simulink library "FUSA_FAULTVAIMAN"  (R2024b)
settings: Solver=VariableStepAuto  StartTime=0.0  StopTime=10.0  RelTol=1e-3
undefined symbols (not defined in the file or in its folder): FUSA_AvailState
libraries: simulink x2
settings Model: Creator=jmbsp  LastModifiedBy=jmbsp

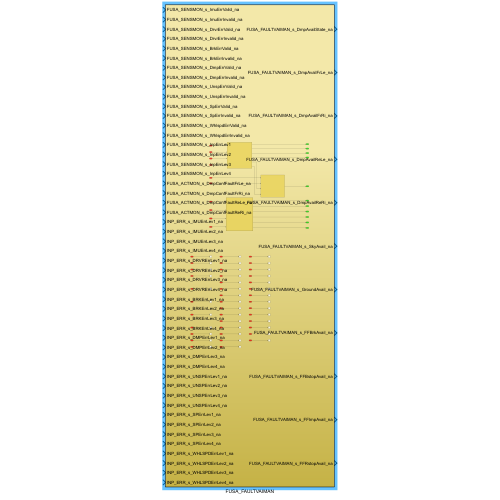
[thumbnail: Simulink's stored preview of the top-level diagram]
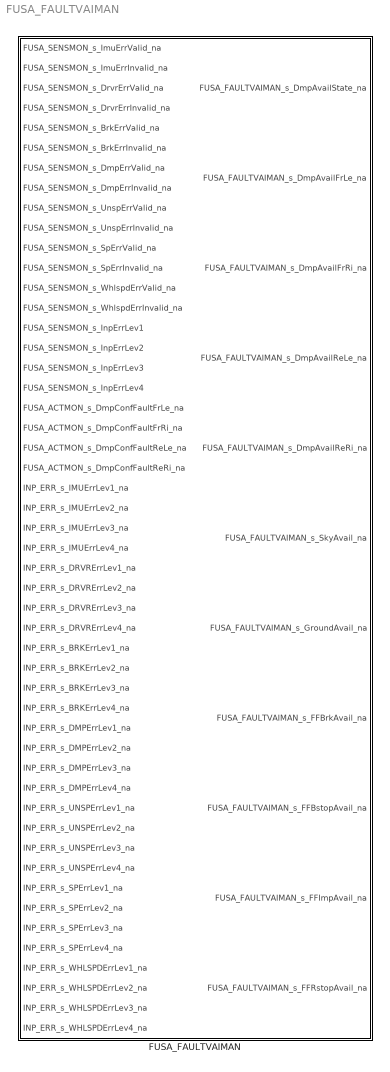
== system FUSA_FAULTVAIMAN ==
  FUSA_FAULTVAIMAN : Subsystem

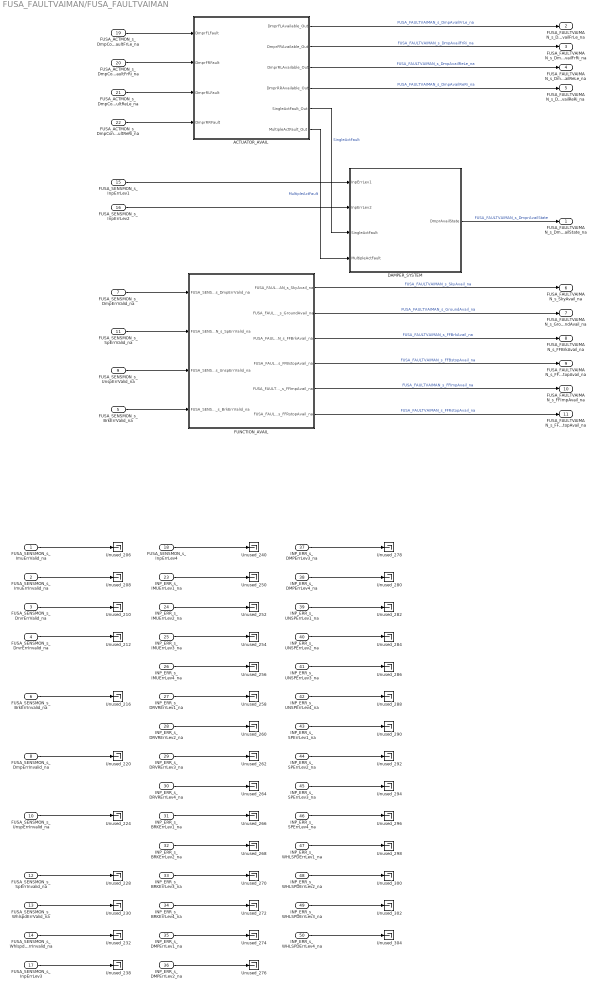
== system FUSA_FAULTVAIMAN/FUSA_FAULTVAIMAN ==
  FUSA_SENSMON_s_ImuErrValid_na : Inport
  FUSA_SENSMON_s_ImuErrInvalid_na : Inport  Port=2
  FUSA_SENSMON_s_DrvrErrValid_na : Inport  Port=3
  FUSA_SENSMON_s_DrvrErrInvalid_na : Inport  Port=4
  FUSA_SENSMON_s_BrkErrValid_na : Inport  Port=5
  FUSA_SENSMON_s_BrkErrInvalid_na : Inport  Port=6
  FUSA_SENSMON_s_DmpErrValid_na : Inport  Port=7
  FUSA_SENSMON_s_DmpErrInvalid_na : Inport  Port=8
  FUSA_SENSMON_s_UnspErrValid_na : Inport  Port=9
  FUSA_SENSMON_s_UnspErrInvalid_na : Inport  Port=10
  FUSA_SENSMON_s_SpErrValid_na : Inport  Port=11
  FUSA_SENSMON_s_SpErrInvalid_na : Inport  Port=12
  FUSA_SENSMON_s_WhlspdErrValid_na : Inport  Port=13
  FUSA_SENSMON_s_WhlspdErrInvalid_na : Inport  Port=14
  FUSA_SENSMON_s_InpErrLev1 : Inport  Port=15  OutDataTypeStr=boolean  PortDimensions=1
  FUSA_SENSMON_s_InpErrLev2 : Inport  Port=16  OutDataTypeStr=boolean  PortDimensions=1
  FUSA_SENSMON_s_InpErrLev3 : Inport  Port=17  OutDataTypeStr=boolean  PortDimensions=1
  FUSA_SENSMON_s_InpErrLev4 : Inport  Port=18  OutDataTypeStr=boolean  PortDimensions=1
  FUSA_ACTMON_s_DmpConfFaultFrLe_na : Inport  Port=19  OutDataTypeStr=boolean  PortDimensions=1
  FUSA_ACTMON_s_DmpConfFaultFrRi_na : Inport  Port=20  OutDataTypeStr=boolean  PortDimensions=1
  FUSA_ACTMON_s_DmpConfFaultReLe_na : Inport  Port=21  OutDataTypeStr=boolean  PortDimensions=1
  FUSA_ACTMON_s_DmpConfFaultReRi_na : Inport  Port=22  OutDataTypeStr=boolean  PortDimensions=1
  INP_ERR_s_IMUErrLev1_na : Inport  Port=23
  INP_ERR_s_IMUErrLev2_na : Inport  Port=24
  INP_ERR_s_IMUErrLev3_na : Inport  Port=25
  INP_ERR_s_IMUErrLev4_na : Inport  Port=26
  INP_ERR_s_DRVRErrLev1_na : Inport  Port=27
  INP_ERR_s_DRVRErrLev2_na : Inport  Port=28
  INP_ERR_s_DRVRErrLev3_na : Inport  Port=29
  INP_ERR_s_DRVRErrLev4_na : Inport  Port=30
  INP_ERR_s_BRKErrLev1_na : Inport  Port=31
  INP_ERR_s_BRKErrLev2_na : Inport  Port=32
  INP_ERR_s_BRKErrLev3_na : Inport  Port=33
  INP_ERR_s_BRKErrLev4_na : Inport  Port=34
  INP_ERR_s_DMPErrLev1_na : Inport  Port=35
  INP_ERR_s_DMPErrLev2_na : Inport  Port=36
  INP_ERR_s_DMPErrLev3_na : Inport  Port=37
  INP_ERR_s_DMPErrLev4_na : Inport  Port=38
  INP_ERR_s_UNSPErrLev1_na : Inport  Port=39
  INP_ERR_s_UNSPErrLev2_na : Inport  Port=40
  INP_ERR_s_UNSPErrLev3_na : Inport  Port=41
  INP_ERR_s_UNSPErrLev4_na : Inport  Port=42
  INP_ERR_s_SPErrLev1_na : Inport  Port=43
  INP_ERR_s_SPErrLev2_na : Inport  Port=44
  INP_ERR_s_SPErrLev3_na : Inport  Port=45
  INP_ERR_s_SPErrLev4_na : Inport  Port=46
  INP_ERR_s_WHLSPDErrLev1_na : Inport  Port=47
  INP_ERR_s_WHLSPDErrLev2_na : Inport  Port=48
  INP_ERR_s_WHLSPDErrLev3_na : Inport  Port=49
  INP_ERR_s_WHLSPDErrLev4_na : Inport  Port=50
  ACTUATOR_AVAIL : Subsystem
  DAMPER_SYSTEM : Subsystem
  FUNCTION_AVAIL : Subsystem
  Unused_{206,208,210,212,216,220,224,228,230,232,238,240,250,252,254,256,258,260,262,264,266,268,270,272,274,276,278,280,282,284,286,288,290,292,294,296,298,300,302,304} (40 alike) : Terminator
  FUSA_FAULTVAIMAN_s_DmpAvailState_na : Outport  OutDataTypeStr=Enum: FUSA_AvailState
  FUSA_FAULTVAIMAN_s_DmpAvailFrLe_na : Outport  Port=2  OutDataTypeStr=boolean
  FUSA_FAULTVAIMAN_s_DmpAvailFrRi_na : Outport  Port=3  OutDataTypeStr=boolean
  FUSA_FAULTVAIMAN_s_DmpAvailReLe_na : Outport  Port=4  OutDataTypeStr=boolean
  FUSA_FAULTVAIMAN_s_DmpAvailReRi_na : Outport  Port=5  OutDataTypeStr=boolean
  FUSA_FAULTVAIMAN_s_SkyAvail_na : Outport  Port=6  OutDataTypeStr=boolean
  FUSA_FAULTVAIMAN_s_GroundAvail_na : Outport  Port=7  OutDataTypeStr=boolean
  FUSA_FAULTVAIMAN_s_FFBrkAvail_na : Outport  Port=8  OutDataTypeStr=boolean
  FUSA_FAULTVAIMAN_s_FFBstopAvail_na : Outport  Port=9  OutDataTypeStr=boolean
  FUSA_FAULTVAIMAN_s_FFImpAvail_na : Outport  Port=10  OutDataTypeStr=boolean
  FUSA_FAULTVAIMAN_s_FFRstopAvail_na : Outport  Port=11  OutDataTypeStr=boolean
  wires:
  FUSA_ACTMON_s_DmpConfFaultFrLe_na/1 -> ACTUATOR_AVAIL/1(DmprFLFault)
  ACTUATOR_AVAIL/1(DmprFLAvailable_Out) -> FUSA_FAULTVAIMAN_s_DmpAvailFrLe_na/1  "FUSA_FAULTVAIMAN_s_DmpAvailFrLe_na"
  FUSA_ACTMON_s_DmpConfFaultFrRi_na/1 -> ACTUATOR_AVAIL/2(DmprFRFault)
  ACTUATOR_AVAIL/2(DmprFRAvailable_Out) -> FUSA_FAULTVAIMAN_s_DmpAvailFrRi_na/1  "FUSA_FAULTVAIMAN_s_DmpAvailFrRi_na"
  FUSA_ACTMON_s_DmpConfFaultReLe_na/1 -> ACTUATOR_AVAIL/3(DmprRLFault)
  ACTUATOR_AVAIL/3(DmprRLAvailable_Out) -> FUSA_FAULTVAIMAN_s_DmpAvailReLe_na/1  "FUSA_FAULTVAIMAN_s_DmpAvailReLe_na"
  FUSA_ACTMON_s_DmpConfFaultReRi_na/1 -> ACTUATOR_AVAIL/4(DmprRRFault)
  ACTUATOR_AVAIL/4(DmprRRAvailable_Out) -> FUSA_FAULTVAIMAN_s_DmpAvailReRi_na/1  "FUSA_FAULTVAIMAN_s_DmpAvailReRi_na"
  FUSA_SENSMON_s_InpErrLev1/1 -> DAMPER_SYSTEM/1(InpErrLev1)
  FUSA_SENSMON_s_InpErrLev2/1 -> DAMPER_SYSTEM/2(InpErrLev2)
  ACTUATOR_AVAIL/5(SingleActFault_Out) -> DAMPER_SYSTEM/3(SingleActFault)  "SingleActFault"
  ACTUATOR_AVAIL/6(MultipleActFault_Out) -> DAMPER_SYSTEM/4(MultipleActFault)  "MultipleActFault"
  DAMPER_SYSTEM/1(DmprAvailState) -> FUSA_FAULTVAIMAN_s_DmpAvailState_na/1  "FUSA_FAULTVAIMAN_s_DmprAvailState"
  FUSA_SENSMON_s_ImuErrValid_na/1 -> Unused_206/1
  FUSA_SENSMON_s_ImuErrInvalid_na/1 -> Unused_208/1
  FUSA_SENSMON_s_DrvrErrValid_na/1 -> Unused_210/1
  FUSA_SENSMON_s_DrvrErrInvalid_na/1 -> Unused_212/1
  FUSA_SENSMON_s_BrkErrInvalid_na/1 -> Unused_216/1
  FUSA_SENSMON_s_DmpErrInvalid_na/1 -> Unused_220/1
  FUSA_SENSMON_s_UnspErrInvalid_na/1 -> Unused_224/1
  FUSA_SENSMON_s_SpErrInvalid_na/1 -> Unused_228/1
  FUSA_SENSMON_s_WhlspdErrValid_na/1 -> Unused_230/1
  FUSA_SENSMON_s_WhlspdErrInvalid_na/1 -> Unused_232/1
  FUSA_SENSMON_s_InpErrLev3/1 -> Unused_238/1
  FUSA_SENSMON_s_InpErrLev4/1 -> Unused_240/1
  INP_ERR_s_IMUErrLev1_na/1 -> Unused_250/1
  INP_ERR_s_IMUErrLev2_na/1 -> Unused_252/1
  INP_ERR_s_IMUErrLev3_na/1 -> Unused_254/1
  INP_ERR_s_IMUErrLev4_na/1 -> Unused_256/1
  INP_ERR_s_DRVRErrLev1_na/1 -> Unused_258/1
  INP_ERR_s_DRVRErrLev2_na/1 -> Unused_260/1
  INP_ERR_s_DRVRErrLev3_na/1 -> Unused_262/1
  INP_ERR_s_DRVRErrLev4_na/1 -> Unused_264/1
  INP_ERR_s_BRKErrLev1_na/1 -> Unused_266/1
  INP_ERR_s_BRKErrLev2_na/1 -> Unused_268/1
  INP_ERR_s_BRKErrLev3_na/1 -> Unused_270/1
  INP_ERR_s_BRKErrLev4_na/1 -> Unused_272/1
  INP_ERR_s_DMPErrLev1_na/1 -> Unused_274/1
  INP_ERR_s_DMPErrLev2_na/1 -> Unused_276/1
  INP_ERR_s_DMPErrLev3_na/1 -> Unused_278/1
  INP_ERR_s_DMPErrLev4_na/1 -> Unused_280/1
  INP_ERR_s_UNSPErrLev1_na/1 -> Unused_282/1
  INP_ERR_s_UNSPErrLev2_na/1 -> Unused_284/1
  INP_ERR_s_UNSPErrLev3_na/1 -> Unused_286/1
  INP_ERR_s_UNSPErrLev4_na/1 -> Unused_288/1
  INP_ERR_s_SPErrLev1_na/1 -> Unused_290/1
  INP_ERR_s_SPErrLev2_na/1 -> Unused_292/1
  INP_ERR_s_SPErrLev3_na/1 -> Unused_294/1
  INP_ERR_s_SPErrLev4_na/1 -> Unused_296/1
  INP_ERR_s_WHLSPDErrLev1_na/1 -> Unused_298/1
  INP_ERR_s_WHLSPDErrLev2_na/1 -> Unused_300/1
  INP_ERR_s_WHLSPDErrLev3_na/1 -> Unused_302/1
  INP_ERR_s_WHLSPDErrLev4_na/1 -> Unused_304/1
  FUSA_SENSMON_s_DmpErrValid_na/1 -> FUNCTION_AVAIL/1(FUSA_SENSMON_s_DmpErrValid_na)
  FUSA_SENSMON_s_SpErrValid_na/1 -> FUNCTION_AVAIL/2(FUSA_SENSMON_s_SpErrValid_na)
  FUSA_SENSMON_s_UnspErrValid_na/1 -> FUNCTION_AVAIL/3(FUSA_SENSMON_s_UnspErrValid_na)
  FUSA_SENSMON_s_BrkErrValid_na/1 -> FUNCTION_AVAIL/4(FUSA_SENSMON_s_BrkErrValid_na)
  FUNCTION_AVAIL/1(FUSA_FAULTVAIMAN_s_SkyAvail_na) -> FUSA_FAULTVAIMAN_s_SkyAvail_na/1  "FUSA_FAULTVAIMAN_s_SkyAvail_na"
  FUNCTION_AVAIL/2(FUSA_FAULTVAIMAN_s_GroundAvail_na) -> FUSA_FAULTVAIMAN_s_GroundAvail_na/1  "FUSA_FAULTVAIMAN_s_GroundAvail_na"
  FUNCTION_AVAIL/3(FUSA_FAULTVAIMAN_s_FFBrkAvail_na) -> FUSA_FAULTVAIMAN_s_FFBrkAvail_na/1  "FUSA_FAULTVAIMAN_s_FFBrkAvail_na"
  FUNCTION_AVAIL/4(FUSA_FAULTVAIMAN_s_FFBstopAvail_na) -> FUSA_FAULTVAIMAN_s_FFBstopAvail_na/1  "FUSA_FAULTVAIMAN_s_FFBstopAvail_na"
  FUNCTION_AVAIL/5(FUSA_FAULTVAIMAN_s_FFImpAvail_na) -> FUSA_FAULTVAIMAN_s_FFImpAvail_na/1  "FUSA_FAULTVAIMAN_s_FFImpAvail_na"
  FUNCTION_AVAIL/6(FUSA_FAULTVAIMAN_s_FFRstopAvail_na) -> FUSA_FAULTVAIMAN_s_FFRstopAvail_na/1  "FUSA_FAULTVAIMAN_s_FFRstopAvail_na"

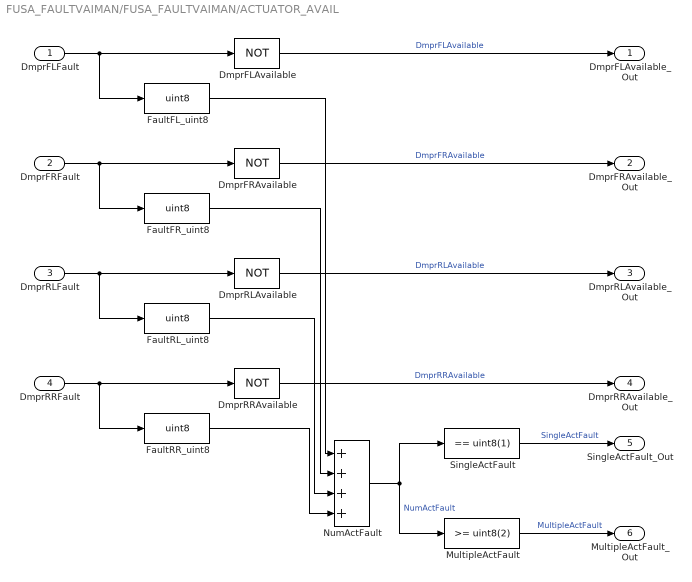
== system FUSA_FAULTVAIMAN/FUSA_FAULTVAIMAN/ACTUATOR_AVAIL ==
  DmprFLFault : Inport  OutDataTypeStr=boolean  PortDimensions=1
  DmprFRFault : Inport  Port=2  OutDataTypeStr=boolean  PortDimensions=1
  DmprRLFault : Inport  Port=3  OutDataTypeStr=boolean  PortDimensions=1
  DmprRRFault : Inport  Port=4  OutDataTypeStr=boolean  PortDimensions=1
  DmprFLAvailable : Logic  Operator=NOT  AllPortsSameDT=off  OutDataTypeStr=boolean
  DmprFRAvailable : Logic  Operator=NOT  AllPortsSameDT=off  OutDataTypeStr=boolean
  DmprRLAvailable : Logic  Operator=NOT  AllPortsSameDT=off  OutDataTypeStr=boolean
  DmprRRAvailable : Logic  Operator=NOT  AllPortsSameDT=off  OutDataTypeStr=boolean
  FaultFL_uint8 : DataTypeConversion  OutDataTypeStr=uint8  SaturateOnIntegerOverflow=off  RndMeth=Floor
  FaultFR_uint8 : DataTypeConversion  OutDataTypeStr=uint8  SaturateOnIntegerOverflow=off  RndMeth=Floor
  FaultRL_uint8 : DataTypeConversion  OutDataTypeStr=uint8  SaturateOnIntegerOverflow=off  RndMeth=Floor
  FaultRR_uint8 : DataTypeConversion  OutDataTypeStr=uint8  SaturateOnIntegerOverflow=off  RndMeth=Floor
  MultipleActFault : simulink/Logic and Bit Operations/Compare To Constant  relop=>=  const=uint8(2)  OutDataTypeStr=boolean
  NumActFault : Sum  Inputs=++++  OutDataTypeStr=uint8  AccumDataTypeStr=uint8
  SingleActFault : simulink/Logic and Bit Operations/Compare To Constant  relop===  const=uint8(1)  OutDataTypeStr=boolean
  DmprFLAvailable_Out : Outport  OutDataTypeStr=boolean
  DmprFRAvailable_Out : Outport  Port=2  OutDataTypeStr=boolean
  DmprRLAvailable_Out : Outport  Port=3  OutDataTypeStr=boolean
  DmprRRAvailable_Out : Outport  Port=4  OutDataTypeStr=boolean
  SingleActFault_Out : Outport  Port=5  OutDataTypeStr=boolean
  MultipleActFault_Out : Outport  Port=6  OutDataTypeStr=boolean
  wires:
  DmprFLFault/1 -> DmprFLAvailable/1, FaultFL_uint8/1
  DmprFLAvailable/1 -> DmprFLAvailable_Out/1  "DmprFLAvailable"
  DmprFRFault/1 -> DmprFRAvailable/1, FaultFR_uint8/1
  DmprFRAvailable/1 -> DmprFRAvailable_Out/1  "DmprFRAvailable"
  DmprRLFault/1 -> DmprRLAvailable/1, FaultRL_uint8/1
  DmprRLAvailable/1 -> DmprRLAvailable_Out/1  "DmprRLAvailable"
  DmprRRFault/1 -> DmprRRAvailable/1, FaultRR_uint8/1
  DmprRRAvailable/1 -> DmprRRAvailable_Out/1  "DmprRRAvailable"
  FaultFL_uint8/1 -> NumActFault/1
  FaultFR_uint8/1 -> NumActFault/2
  FaultRL_uint8/1 -> NumActFault/3
  FaultRR_uint8/1 -> NumActFault/4
  NumActFault/1 -> SingleActFault/1, MultipleActFault/1  "NumActFault"
  SingleActFault/1 -> SingleActFault_Out/1  "SingleActFault"
  MultipleActFault/1 -> MultipleActFault_Out/1  "MultipleActFault"

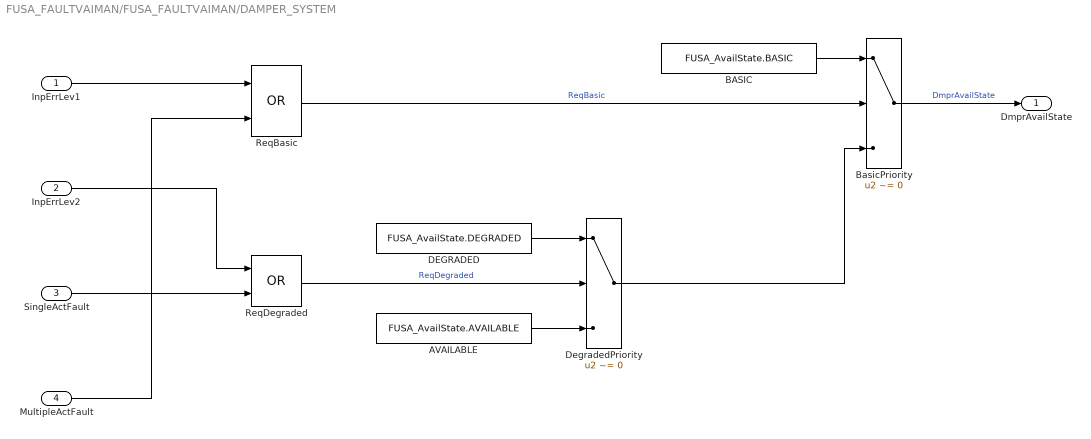
== system FUSA_FAULTVAIMAN/FUSA_FAULTVAIMAN/DAMPER_SYSTEM ==
  InpErrLev1 : Inport  OutDataTypeStr=boolean  PortDimensions=1
  InpErrLev2 : Inport  Port=2  OutDataTypeStr=boolean  PortDimensions=1
  SingleActFault : Inport  Port=3  OutDataTypeStr=boolean  PortDimensions=1
  MultipleActFault : Inport  Port=4  OutDataTypeStr=boolean  PortDimensions=1
  AVAILABLE : Constant  Value=FUSA_AvailState.AVAILABLE  OutDataTypeStr=Enum: FUSA_AvailState
  BASIC : Constant  Value=FUSA_AvailState.BASIC  OutDataTypeStr=Enum: FUSA_AvailState
  BasicPriority : Switch  Criteria=u2 ~= 0  SaturateOnIntegerOverflow=off  InputSameDT=off
  DEGRADED : Constant  Value=FUSA_AvailState.DEGRADED  OutDataTypeStr=Enum: FUSA_AvailState
  DegradedPriority : Switch  Criteria=u2 ~= 0  SaturateOnIntegerOverflow=off  InputSameDT=off
  ReqBasic : Logic  Operator=OR  AllPortsSameDT=off  OutDataTypeStr=boolean
  ReqDegraded : Logic  Operator=OR  AllPortsSameDT=off  OutDataTypeStr=boolean
  DmprAvailState : Outport  OutDataTypeStr=Enum: FUSA_AvailState
  wires:
  InpErrLev1/1 -> ReqBasic/1
  MultipleActFault/1 -> ReqBasic/2
  InpErrLev2/1 -> ReqDegraded/1
  SingleActFault/1 -> ReqDegraded/2
  DEGRADED/1 -> DegradedPriority/1
  ReqDegraded/1 -> DegradedPriority/2  "ReqDegraded"
  AVAILABLE/1 -> DegradedPriority/3
  BASIC/1 -> BasicPriority/1
  ReqBasic/1 -> BasicPriority/2  "ReqBasic"
  DegradedPriority/1 -> BasicPriority/3
  BasicPriority/1 -> DmprAvailState/1  "DmprAvailState"

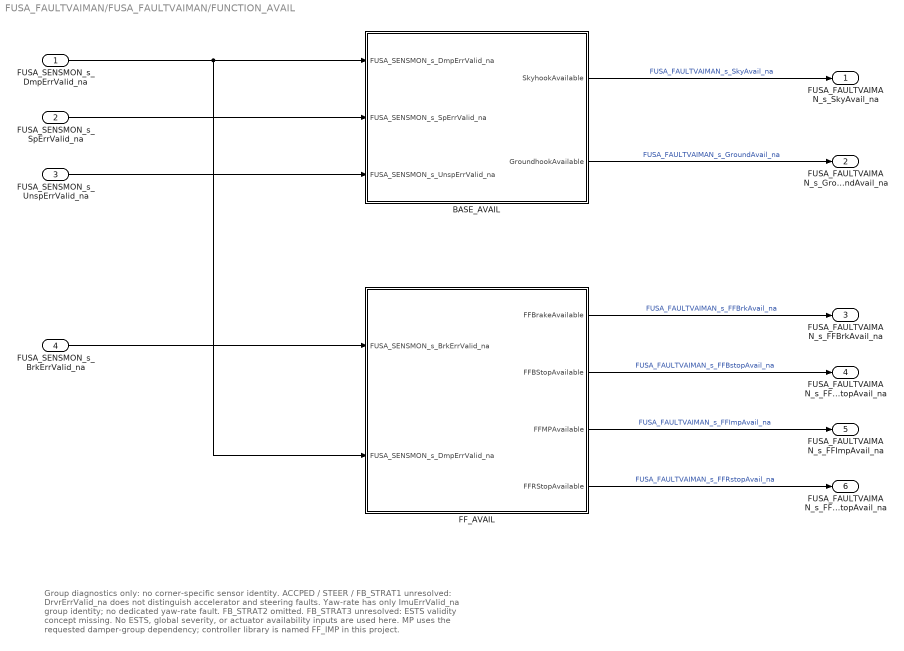
== system FUSA_FAULTVAIMAN/FUSA_FAULTVAIMAN/FUNCTION_AVAIL ==
  note: Group diagnostics only: no corner-specific sensor identity.
      | ACCPED / STEER / FB_STRAT1 unresolved: DrvrErrValid_na does not distinguish accelerator and steering faults.
      | Yaw-rate has only ImuErrValid_na group identity; no dedicated yaw-rate fault.
      | FB_STRAT2 omitted. FB_STRAT3 unresolved: ESTS validity concept missing.
      | No ESTS, global severity, or actuator availability inputs are used here.
      | MP uses the requested damper-group dependency; controller library is named FF_IMP in this project.
  FUSA_SENSMON_s_DmpErrValid_na : Inport
  FUSA_SENSMON_s_SpErrValid_na : Inport  Port=2
  FUSA_SENSMON_s_UnspErrValid_na : Inport  Port=3
  FUSA_SENSMON_s_BrkErrValid_na : Inport  Port=4
  BASE_AVAIL : Subsystem
  FF_AVAIL : Subsystem
  FUSA_FAULTVAIMAN_s_SkyAvail_na : Outport  OutDataTypeStr=boolean
  FUSA_FAULTVAIMAN_s_GroundAvail_na : Outport  Port=2  OutDataTypeStr=boolean
  FUSA_FAULTVAIMAN_s_FFBrkAvail_na : Outport  Port=3  OutDataTypeStr=boolean
  FUSA_FAULTVAIMAN_s_FFBstopAvail_na : Outport  Port=4  OutDataTypeStr=boolean
  FUSA_FAULTVAIMAN_s_FFImpAvail_na : Outport  Port=5  OutDataTypeStr=boolean
  FUSA_FAULTVAIMAN_s_FFRstopAvail_na : Outport  Port=6  OutDataTypeStr=boolean
  wires:
  FUSA_SENSMON_s_DmpErrValid_na/1 -> BASE_AVAIL/1(FUSA_SENSMON_s_DmpErrValid_na), FF_AVAIL/2(FUSA_SENSMON_s_DmpErrValid_na)
  FUSA_SENSMON_s_SpErrValid_na/1 -> BASE_AVAIL/2(FUSA_SENSMON_s_SpErrValid_na)
  FUSA_SENSMON_s_UnspErrValid_na/1 -> BASE_AVAIL/3(FUSA_SENSMON_s_UnspErrValid_na)
  FUSA_SENSMON_s_BrkErrValid_na/1 -> FF_AVAIL/1(FUSA_SENSMON_s_BrkErrValid_na)
  BASE_AVAIL/1(SkyhookAvailable) -> FUSA_FAULTVAIMAN_s_SkyAvail_na/1  "FUSA_FAULTVAIMAN_s_SkyAvail_na"
  BASE_AVAIL/2(GroundhookAvailable) -> FUSA_FAULTVAIMAN_s_GroundAvail_na/1  "FUSA_FAULTVAIMAN_s_GroundAvail_na"
  FF_AVAIL/1(FFBrakeAvailable) -> FUSA_FAULTVAIMAN_s_FFBrkAvail_na/1  "FUSA_FAULTVAIMAN_s_FFBrkAvail_na"
  FF_AVAIL/2(FFBStopAvailable) -> FUSA_FAULTVAIMAN_s_FFBstopAvail_na/1  "FUSA_FAULTVAIMAN_s_FFBstopAvail_na"
  FF_AVAIL/3(FFMPAvailable) -> FUSA_FAULTVAIMAN_s_FFImpAvail_na/1  "FUSA_FAULTVAIMAN_s_FFImpAvail_na"
  FF_AVAIL/4(FFRStopAvailable) -> FUSA_FAULTVAIMAN_s_FFRstopAvail_na/1  "FUSA_FAULTVAIMAN_s_FFRstopAvail_na"

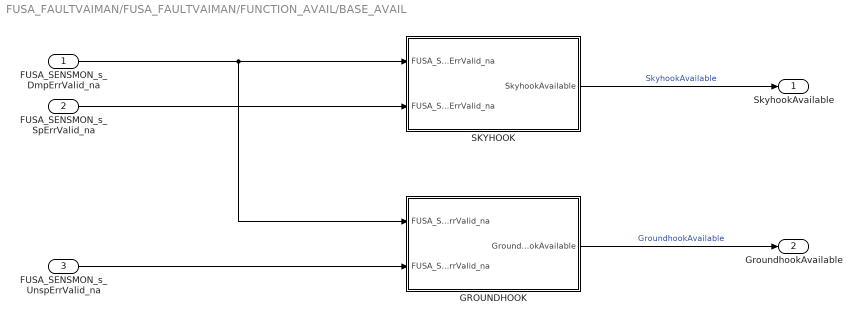
== system FUSA_FAULTVAIMAN/FUSA_FAULTVAIMAN/FUNCTION_AVAIL/BASE_AVAIL ==
  FUSA_SENSMON_s_DmpErrValid_na : Inport
  FUSA_SENSMON_s_SpErrValid_na : Inport  Port=2
  FUSA_SENSMON_s_UnspErrValid_na : Inport  Port=3
  GROUNDHOOK : Subsystem
  SKYHOOK : Subsystem
  SkyhookAvailable : Outport  OutDataTypeStr=boolean
  GroundhookAvailable : Outport  Port=2  OutDataTypeStr=boolean
  wires:
  FUSA_SENSMON_s_DmpErrValid_na/1 -> SKYHOOK/1(FUSA_SENSMON_s_DmpErrValid_na), GROUNDHOOK/1(FUSA_SENSMON_s_DmpErrValid_na)
  FUSA_SENSMON_s_SpErrValid_na/1 -> SKYHOOK/2(FUSA_SENSMON_s_SpErrValid_na)
  SKYHOOK/1(SkyhookAvailable) -> SkyhookAvailable/1  "SkyhookAvailable"
  FUSA_SENSMON_s_UnspErrValid_na/1 -> GROUNDHOOK/2(FUSA_SENSMON_s_UnspErrValid_na)
  GROUNDHOOK/1(GroundhookAvailable) -> GroundhookAvailable/1  "GroundhookAvailable"

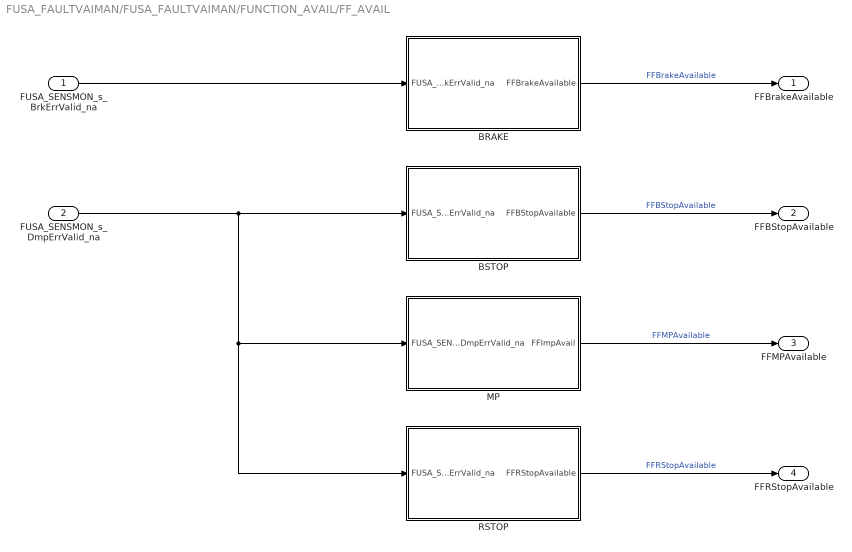
== system FUSA_FAULTVAIMAN/FUSA_FAULTVAIMAN/FUNCTION_AVAIL/FF_AVAIL ==
  FUSA_SENSMON_s_BrkErrValid_na : Inport
  FUSA_SENSMON_s_DmpErrValid_na : Inport  Port=2
  BRAKE : Subsystem
  BSTOP : Subsystem
  MP : Subsystem
  RSTOP : Subsystem
  FFBrakeAvailable : Outport  OutDataTypeStr=boolean
  FFBStopAvailable : Outport  Port=2  OutDataTypeStr=boolean
  FFMPAvailable : Outport  Port=3  OutDataTypeStr=boolean
  FFRStopAvailable : Outport  Port=4  OutDataTypeStr=boolean
  wires:
  FUSA_SENSMON_s_BrkErrValid_na/1 -> BRAKE/1(FUSA_SENSMON_s_BrkErrValid_na)
  BRAKE/1(FFBrakeAvailable) -> FFBrakeAvailable/1  "FFBrakeAvailable"
  FUSA_SENSMON_s_DmpErrValid_na/1 -> MP/1(FUSA_SENSMON_s_DmpErrValid_na), RSTOP/1(FUSA_SENSMON_s_DmpErrValid_na), BSTOP/1(FUSA_SENSMON_s_DmpErrValid_na)
  BSTOP/1(FFBStopAvailable) -> FFBStopAvailable/1  "FFBStopAvailable"
  MP/1(FFImpAvail) -> FFMPAvailable/1  "FFMPAvailable"
  RSTOP/1(FFRStopAvailable) -> FFRStopAvailable/1  "FFRStopAvailable"

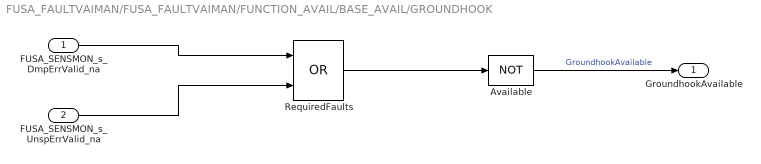
== system FUSA_FAULTVAIMAN/FUSA_FAULTVAIMAN/FUNCTION_AVAIL/BASE_AVAIL/GROUNDHOOK ==
  FUSA_SENSMON_s_DmpErrValid_na : Inport
  FUSA_SENSMON_s_UnspErrValid_na : Inport  Port=2
  Available : Logic  Operator=NOT  AllPortsSameDT=off  OutDataTypeStr=boolean
  RequiredFaults : Logic  Operator=OR  AllPortsSameDT=off  OutDataTypeStr=boolean
  GroundhookAvailable : Outport  OutDataTypeStr=boolean
  wires:
  FUSA_SENSMON_s_DmpErrValid_na/1 -> RequiredFaults/1
  FUSA_SENSMON_s_UnspErrValid_na/1 -> RequiredFaults/2
  RequiredFaults/1 -> Available/1
  Available/1 -> GroundhookAvailable/1  "GroundhookAvailable"

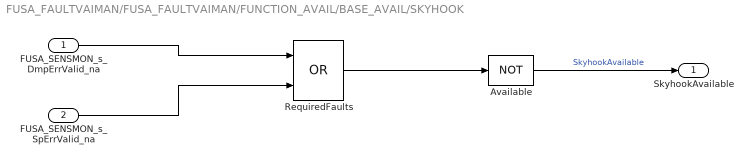
== system FUSA_FAULTVAIMAN/FUSA_FAULTVAIMAN/FUNCTION_AVAIL/BASE_AVAIL/SKYHOOK ==
  FUSA_SENSMON_s_DmpErrValid_na : Inport
  FUSA_SENSMON_s_SpErrValid_na : Inport  Port=2
  Available : Logic  Operator=NOT  AllPortsSameDT=off  OutDataTypeStr=boolean
  RequiredFaults : Logic  Operator=OR  AllPortsSameDT=off  OutDataTypeStr=boolean
  SkyhookAvailable : Outport  OutDataTypeStr=boolean
  wires:
  FUSA_SENSMON_s_DmpErrValid_na/1 -> RequiredFaults/1
  FUSA_SENSMON_s_SpErrValid_na/1 -> RequiredFaults/2
  RequiredFaults/1 -> Available/1
  Available/1 -> SkyhookAvailable/1  "SkyhookAvailable"

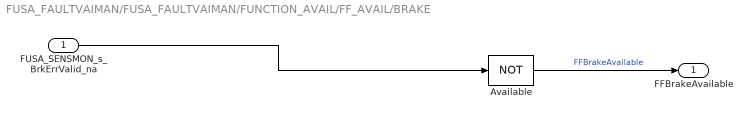
== system FUSA_FAULTVAIMAN/FUSA_FAULTVAIMAN/FUNCTION_AVAIL/FF_AVAIL/BRAKE ==
  FUSA_SENSMON_s_BrkErrValid_na : Inport
  Available : Logic  Operator=NOT  AllPortsSameDT=off  OutDataTypeStr=boolean
  FFBrakeAvailable : Outport  OutDataTypeStr=boolean
  wires:
  FUSA_SENSMON_s_BrkErrValid_na/1 -> Available/1
  Available/1 -> FFBrakeAvailable/1  "FFBrakeAvailable"

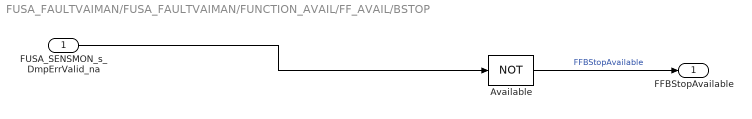
== system FUSA_FAULTVAIMAN/FUSA_FAULTVAIMAN/FUNCTION_AVAIL/FF_AVAIL/BSTOP ==
  FUSA_SENSMON_s_DmpErrValid_na : Inport
  Available : Logic  Operator=NOT  AllPortsSameDT=off  OutDataTypeStr=boolean
  FFBStopAvailable : Outport  OutDataTypeStr=boolean
  wires:
  FUSA_SENSMON_s_DmpErrValid_na/1 -> Available/1
  Available/1 -> FFBStopAvailable/1  "FFBStopAvailable"

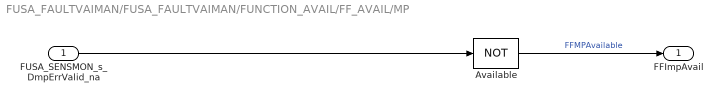
== system FUSA_FAULTVAIMAN/FUSA_FAULTVAIMAN/FUNCTION_AVAIL/FF_AVAIL/MP ==
  FUSA_SENSMON_s_DmpErrValid_na : Inport
  Available : Logic  Operator=NOT  AllPortsSameDT=off  OutDataTypeStr=boolean
  FFImpAvail : Outport  OutDataTypeStr=boolean
  wires:
  FUSA_SENSMON_s_DmpErrValid_na/1 -> Available/1
  Available/1 -> FFImpAvail/1  "FFMPAvailable"

== system FUSA_FAULTVAIMAN/FUSA_FAULTVAIMAN/FUNCTION_AVAIL/FF_AVAIL/RSTOP ==
  FUSA_SENSMON_s_DmpErrValid_na : Inport
  Available : Logic  Operator=NOT  AllPortsSameDT=off  OutDataTypeStr=boolean
  FFRStopAvailable : Outport  OutDataTypeStr=boolean
  wires:
  FUSA_SENSMON_s_DmpErrValid_na/1 -> Available/1
  Available/1 -> FFRStopAvailable/1  "FFRStopAvailable"
